simulink model "pr632_loop_filter"  (R2018b)
settings: Solver=VariableStepAuto  StartTime=0.0  StopTime=1000/fs  RelTol=1e-3  EnableMultiTasking=on
PreLoadFcn:
  | fs=100e6;
libraries: dspsrcs4 x1
CloseFcn:
  | clear all;
settings Model: Creator=GRIHA  LastModifiedBy=Григорий Фокин
settings DataIOCC: LimitDataPoints=on
settings OptimizationCC: LifeSpan=inf
settings DebuggingCC: AllowSymbolicDim=off  SFUnexpectedBacktrackingDiag=warning  SFNoUnconditionalDefaultTransitionDiag=warning  SFExecutionAtInitializationDiag=none
settings ModelReferenceCC: PropagateSignalLabelsOutOfModel=off
settings SFSimCC: SimUseLocalCustomCode=off
settings RTWCC: RTWUseLocalCustomCode=off
settings CodeAppCC: StateflowObjectComments=on
settings GRTTargetCC: TargetLangStandard=C89/C90 (ANSI)
settings ConfigComp: CovMetricSettings=dw  CovHtmlReporting=on  CovSaveCumulativeToWorkspaceVar=on  CovSaveSingleToWorkspaceVar=on  CovExternalEMLEnable=off

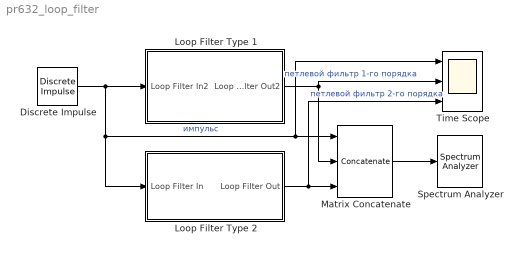
== system pr632_loop_filter ==
  Discrete Impulse : dspsrcs4/Discrete  Impulse  Delay=0  SampleTime=1/fs  FrameSample=1  OutputFrames=off  dataType=double  isSigned=on  wordLen=16  udDataType=sfix(16)  fracBitsMode=Best precision  numFracBits=15  OutDataTypeStr=double  LastOutDataTypeStr=double
  Loop Filter Type 1 : Subsystem  mask{K1=0.03125}
      mask prompts: K1 "K1 (proportional path)"
  Loop Filter Type 2 : Subsystem  mask{K1=0.03125, K2=1.25e-4}
      mask prompts: K1 "K1 (proportional path)"; K2 "K2 (integral path)"
  Matrix Concatenate : Concatenate  NumInputs=3  Mode=Multidimensional array  ConcatenateDimension=2
  Spectrum Analyzer : SpectrumAnalyzer
  Time Scope : Scope  NumInputPorts=3
  wires:
  Discrete Impulse/1 -> Loop Filter Type 1/1(Loop Filter In2), Loop Filter Type 2/1(Loop Filter In), Time Scope/1, Matrix Concatenate/1  "импульс"
  Loop Filter Type 1/1(Loop Filter Out2) -> Time Scope/2, Matrix Concatenate/2  "петлевой фильтр 1-го порядка"
  Loop Filter Type 2/1(Loop Filter Out) -> Time Scope/3, Matrix Concatenate/3  "петлевой фильтр 2-го порядка"
  Matrix Concatenate/1 -> Spectrum Analyzer/1

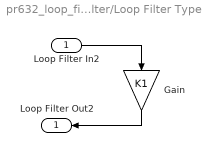
== system pr632_loop_filter/Loop Filter Type 1 ==
  Loop Filter In2 : Inport
  Gain : Gain  Gain=K1
  Loop Filter Out2 : Outport
  wires:
  Loop Filter In2/1 -> Gain/1
  Gain/1 -> Loop Filter Out2/1

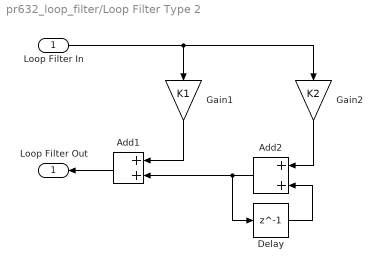
== system pr632_loop_filter/Loop Filter Type 2 ==
  Loop Filter In : Inport
  Add1 : Sum
  Add2 : Sum
  Delay : Delay  DelayLength=1  InitialCondition=0
  Gain1 : Gain  Gain=K1
  Gain2 : Gain  Gain=K2
  Loop Filter Out : Outport
  wires:
  Loop Filter In/1 -> Gain2/1, Gain1/1
  Add1/1 -> Loop Filter Out/1
  Gain1/1 -> Add1/1
  Add2/1 -> Delay/1, Add1/2
  Gain2/1 -> Add2/1
  Delay/1 -> Add2/2
